simulink model "Cognata_Amp_Tobi_split1"  (R2020a)
settings: Solver=ode45  StartTime=0.0  StopTime=inf  RelTol=1e-3
model workspace (MAT data in the model file):
  cfg_native : object (value not decoded)
  en_add_channels = 1
  host_ip = 2130706433
  host_port = 50223
  local_ip = 2130706433
  local_port = 50224
  num_en_channels = 32
  num_samples = 1
  sample_rate = 250
  serial_number = 'NB-2015.10.93'
undefined symbols (not defined in the file or in its folder): A1, A104210, A138674, A141395, A30722, C1, C30722, currentCFG_Cognata_Amp_Tobi_split_UB, D1, D104210, I1, J138674, O141395, UB, W1, W104210
libraries: robotlib x18, gtecHighspeedLib x16, dspstat3 x2, simulink x2, TobiiEyeTrackerLib x1, gUSBamplib x1
settings Model: ModifiedByFormat=g.tec  Creator=g.tec medical engineering  LastModifiedBy=g.tec
settings DataIOCC: LimitDataPoints=on  SaveFormat=Array  ReturnWorkspaceOutputs=off
settings OptimizationCC: BlockReduction=off  BooleanDataType=off  LifeSpan=inf
settings DebuggingCC: SaveWithParameterizedLinksMsg=none  UnderspecifiedInitializationDetection=Classic  MergeDetectMultiDrivingBlocksExec=none  SignalResolutionControl=TryResolveAllWithWarning  FrameProcessingCompatibilityMsg=none  SFUnexpectedBacktrackingDiag=warning  SFNoUnconditionalDefaultTransitionDiag=warning  SFExecutionAtInitializationDiag=none  ArithmeticOperatorsInVariantConditions=warning
settings HardwareCC: ProdBitPerPointer=32  ProdBitPerSizeT=32  ProdBitPerPtrDiffT=32  ProdLargestAtomicFloat=None  ProdIntDivRoundTo=Undefined  ProdEndianess=Unspecified  ProdWordSize=32  ProdHWDeviceType=32-bit Generic  TargetUnknown=on
settings ModelReferenceCC: PropagateSignalLabelsOutOfModel=off
settings SFSimCC: SimUseLocalCustomCode=off  CustomCodeUndefinedFunction=UseInterfaceOnly
settings RTWCC: RTWUseLocalCustomCode=off
settings CodeAppCC: StateflowObjectComments=on
settings GRTTargetCC: TargetLangStandard=C89/C90 (ANSI)
settings ConfigComp: CovMetricSettings=dw  CovHtmlReporting=on  CovSaveCumulativeToWorkspaceVar=on  CovSaveSingleToWorkspaceVar=on  CovExternalEMLEnable=off

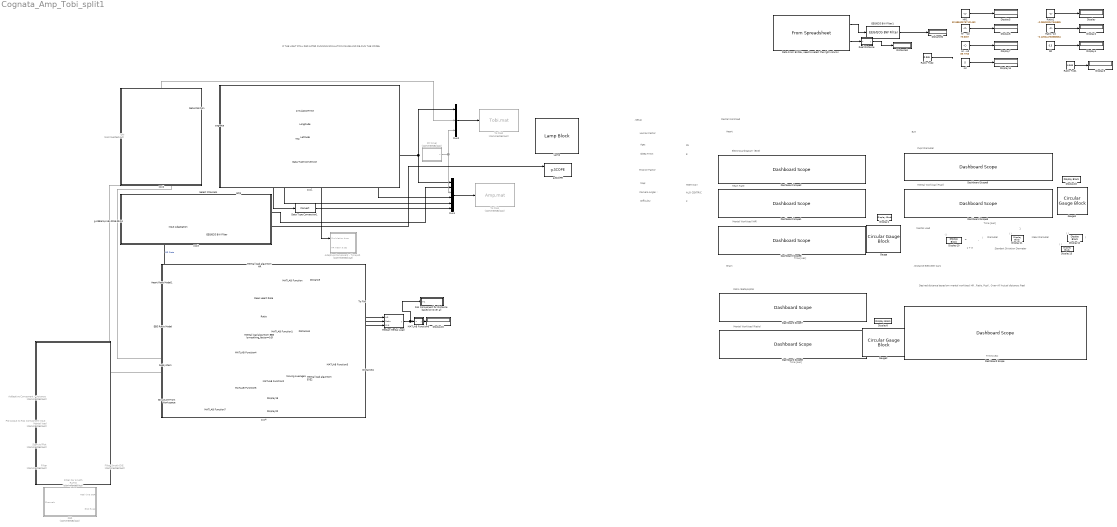
== system Cognata_Amp_Tobi_split1 ==
  note: Mental Load
  note: IF THE LIGHT STILL RED AFTER
      | RUNNING SIMULATION PAUSE AND RE-RUN THE MODEL
  note: Mission Factor
  note: Mental Workload
  note: Difficulty:
  note: Age:
  note: Brain
  note: ALO CENTRIC
  note: . Setup
  note: . Distance Between Cars
  note: Heart
  note: HIGH WAY
  note: Sleep Time:
  note: Camera Angle: :
  note: Human Factor
  note: Map:
  note: Electrocardiogram (ECG)
  note: Mental Workload (HR)
  note: Heart Rate
  note: Ratio (Beta/Alpha)
  note: Time [sec]
  note: Mental Workload (Ratio)
  note: Desired distance based om mental worklaod:
      | HR , Ratio, Pupil , Over-All
      |
      | Actual distance: Real
  note: Time [sec]
  note: 25
  note: 8
  note: 2
  note: Eye
  note: Pupil Diameter
  note: Mental Workload (Pupil)
  note: Time [sec]
  note: Time [sec]
  note: ( )
  note: 1
  note: Diameter
  note: ( )
  note: Mean Diameter
  note: ( )
  note: Standart Diviation Diameter
  note: ( )
  note: 1 + e
  note: (
  note: )
  note: -
  note: =
  "Adaptive Component - Time/HR " : Subsystem  Commented=on
  Addaptive Component - Distance : Subsystem  Commented=on
  Dashboard Scope : DashboardScope  ShowInitialText=off  TimeSpan=10  Ymin=-1  Ymax=20  LegendPosition=Hide  ScaleAtStop=off
  Dashboard Scope1 : DashboardScope  TimeSpan=10  Ymin=0  Ymax=100  LegendPosition=Hide  ScaleAtStop=off
  Dashboard Scope2 : DashboardScope  TimeSpan=10  Ymin=-3000  Ymax=1000  LegendPosition=Hide  ScaleAtStop=off
  Dashboard Scope3 : DashboardScope  TimeSpan=10  Ymin=0  Ymax=1  LegendPosition=Hide  ScaleAtStop=off
  Dashboard Scope6 : DashboardScope  TimeSpan=10  Ymin=0  Ymax=1  LegendPosition=Hide  ScaleAtStop=off
  Dashboard Scope7 : DashboardScope  TimeSpan=10  Ymin=0  Ymax=0.5  LegendPosition=Hide  ScaleAtStop=off
  Dashboard Scope8 : DashboardScope  TimeSpan=10  Ymin=0  Ymax=1  LegendPosition=Hide  ScaleAtStop=off
  Dashboard Scope9 : DashboardScope  TimeSpan=10  Ymin=0  Ymax=5  LegendPosition=Hide  ScaleAtStop=off
  "Data From EXCEL, need to select the right column " : FromSpreadsheet  FileName=C:\Users\LAB-OREN3\Desktop\CognataData\Participants_DATA\Test\4\g.techAmp Data of A1_546053_COMBINED_CUBE_DELAY_50_TTC_15 at (12;30;7).xlsx  SheetName=גיליון1  Range=A1:A104210,D1:D104210,W1:W104210  SampleTime=0.001953125
  Data Type Conversion : DataTypeConversion
  Data Type Conversion1 : DataTypeConversion
  Display{,2..7,14..15,19..20} (11 alike) : Display
  Display{1,8,10..11,13,16} (6 alike) : DisplayBlock  LabelPosition=Hide  Format=bank  Transparency=1
  Display12 : DisplayBlock  LabelPosition=Hide  Format=bank  Transparency=1  Layout=Fill available space
  Distance{,1..4} (5 alike) : Display
  ECG : MATLAB Function  TreatAsAtomicUnit=on
  EEG Ratio Model : Subsystem
  EEG/ECG BW Filter : gtecHighspeedLib/EEG//ECG BW Filter  Order=6  LowerFreq=0.1  UpperFreq=30  SampFreq=512
      settings: SourceProductName=g.HIsys Library
  EEG/ECG BW Filter1 : gtecHighspeedLib/EEG//ECG BW Filter  Order=6  LowerFreq=0.1  UpperFreq=30  SampFreq=512
      settings: SourceProductName=g.HIsys Library
  Filter : Subsystem  Commented=on
  Filter For smoth RATIO : Subsystem  Commented=on
  Filter Smoth EYE : Subsystem  Commented=on
  GSR : Subsystem  Commented=on
  Gauge : CircularGaugeBlock  LabelPosition=Hide  ScaleMax=1  TickInterval=0.2
  Gauge1 : CircularGaugeBlock  LabelPosition=Hide  ScaleMax=1  TickInterval=0.2
  Gauge2 : CircularGaugeBlock  LabelPosition=Hide  ScaleMax=1  TickInterval=0.2
  Gaze Position : Display
  HR1 : Constant  Value=82.688405797101450  VectorParams1D=off  SampleTime=0.5
  Heart Rate Model1 : ModelReference  ModelNameDialog=Heart_Rate_Model_Test  SimulationMode=Normal  ModelReferenceVersion=2.18.00
  Hr   -sd : Constant  Value=75.6007  SampleTime=0.5
  Hr - sd : Constant  Value=89.7753  SampleTime=0.5
  Input Adaptation : Subsystem
  Lamp : LampBlock
  Latitude : Display
  Longitude : Display
  MATLAB Function : MATLAB Function  TreatAsAtomicUnit=on
  MATLAB Function1 : MATLAB Function  TreatAsAtomicUnit=on
  MATLAB Function2 : MATLAB Function  TreatAsAtomicUnit=on
  MATLAB Function3 : MATLAB Function  TreatAsAtomicUnit=on
  MATLAB Function4 : MATLAB Function  TreatAsAtomicUnit=on
  MATLAB Function5 : MATLAB Function  TreatAsAtomicUnit=on
  MATLAB Function6 : MATLAB Function  TreatAsAtomicUnit=on
  MATLAB Function7 : MATLAB Function  TreatAsAtomicUnit=on
  "Mean Heart Rate " : Display
  Median Mental Load : MATLAB Function  TreatAsAtomicUnit=on
  "Mental load alguritom EEG (smoothing_factor=0.5) " : MATLAB Function  TreatAsAtomicUnit=on
  Mental load alguritom EYE2 : MATLAB Function  TreatAsAtomicUnit=on
  Mental load alguritom HR : MATLAB Function  TreatAsAtomicUnit=on
  Moving Average1 : dspstat3/Moving Average  Method=Sliding window  ForgettingFactorPort=off  SpecifyWindowLength=on  WindowLength=512  ForgettingFactor=0.9  SimulateUsing=Code generation
  Mux1 : Mux  Inputs=6
  Mux2 : Mux  Inputs=3
  PC timer : MATLAB Function  Commented=on  TreatAsAtomicUnit=on
  PID output to Ros Component input Mental load : Subsystem  Commented=on
  Ratio : Display
  Ratio +sd1 : Constant  Value=4.644  SampleTime=0.5
  Ratio +sd2 : Constant  Value=0.345  SampleTime=0.5
  Ratio -sd : Constant  Value=-0.125044783588084  SampleTime=0.5
  Ratio1 : Constant  Value=-0.086230047345885  VectorParams1D=off  SampleTime=0.5
  Real Distance : MATLAB Function  TreatAsAtomicUnit=on
  Ros Component for Distance based on Over all : Subsystem
  SD : Constant  Value=0.3  SampleTime=0.5
  Select Channels : gtecHighspeedLib/Select Channels  selectedchannels=[2]  totalchannels=14
      settings: SourceProductName=g.HIsys Library
  Sigmuid Plot : MATLAB Function  Commented=on  TreatAsAtomicUnit=on
  Structure From Workspace : FromWorkspace  VariableName=wave
  Subsystem : Subsystem
  TTC : Display
  To File : ToFile  Filename=Avrage.mat  MatrixName=Avrage
  To File1 : ToFile  Commented=on  Filename=Amp.mat  MatrixName=Ampdata
  To File2 : ToFile  Commented=on  Filename=Tobi.mat  MatrixName=Tobidata
  Tobi : Subsystem  Commented=on
  cognata : Subsystem
  g.SCOPE : gtecHighspeedLib/g.SCOPE
      settings: SourceProductName=g.HIsys Library
  g.USBamp UB-2015.09.13 : gUSBamplib/g.USBamp  cfg=currentCFG_Cognata_Amp_Tobi_split_UB-2015.09.13.cfg  snr=UB-2015.09.13
      settings: SourceProductName=g.USBamp
  sd : Constant  Value=5  SampleTime=0.5
  simulationTime : Display
  zzz1 : Subsystem  TreatAsAtomicUnit=on
      settings: OpenFcn=% no-op
      mask Display: disp('')
  zzz2 : Subsystem  TreatAsAtomicUnit=on
      settings: OpenFcn=% no-op
      mask Display: disp('')
  zzz3 : Subsystem  TreatAsAtomicUnit=on
      settings: OpenFcn=% no-op
      mask Display: disp('')
  zzz4 : Subsystem  TreatAsAtomicUnit=on
      settings: OpenFcn=% no-op
      mask Display: disp('')
  zzz5 : Subsystem  TreatAsAtomicUnit=on
      settings: OpenFcn=% no-op
      mask Display: disp('')
  wires:
  Tobi/2(Sum) -> Mux2/2
  Input Adaptation/1(Out) -> Mux1/2, EEG/ECG BW Filter/1
  Mux1/1 -> To File1/1
  Data Type Conversion/1 -> Mux2/1, Mux1/1, "Adaptive Component - Time/HR "/1(Simlulation time)
  g.USBamp UB-2015.09.13/1 -> Heart Rate Model1/1, EEG Ratio Model/1(Channels), Input Adaptation/1(In)  "EG Data"
  cognata/1(SimulationTime) -> Data Type Conversion/1, simulationTime/1
  Mux2/1 -> To File2/1
  Tobi/1(Gaze Pos) -> Gaze Position/1
  PC timer/1(z) -> Mux1/3, Mux2/3
  EEG/ECG BW Filter/1 -> Select Channels/1, g.SCOPE/1
  cognata/3(Latitude) -> Mux1/5, Latitude/1
  cognata/4(TTC) -> TTC/1, Data Type Conversion1/1
  cognata/2(Longitude) -> Mux1/4, Longitude/1
  Data Type Conversion1/1 -> Mux1/6
  MATLAB Function/1(y) -> Distance/1
  ECG/1(y) -> ?
  Select Channels/1 -> ECG/1(u)
  Mental load alguritom HR/1(y) -> Median Mental Load/1(HR), To File/1, MATLAB Function/1(u)
  "Mental load alguritom EEG (smoothing_factor=0.5) "/1(y) -> Median Mental Load/2(Ratio), MATLAB Function1/1(u)
  MATLAB Function1/1(y) -> Distance1/1
  "Data From EXCEL, need to select the right column "/1 -> EEG/ECG BW Filter1/1
  EEG/ECG BW Filter1/1 -> Distance2/1
  "Data From EXCEL, need to select the right column "/2 -> Real Distance/1(u)
  Ratio1/1 -> Display/1
  Ratio -sd/1 -> Display2/1
  SD/1 -> Display4/1
  Hr - sd/1 -> Display7/1
  Hr   -sd/1 -> Display6/1
  HR1/1 -> Display5/1
  Real Distance/1(y) -> Distance3/1
  sd/1 -> Display14/1
  Tobi/3(Pupil diameter Right Real-Time) -> Subsystem/1(Pupil diameter Right Real-Time)
  MATLAB Function2/1(y) -> Moving Average1/1
  Mental load alguritom EYE2/1(y) -> Median Mental Load/3(eye), MATLAB Function3/1(u)
  MATLAB Function3/1(y) -> Distance4/1
  Moving Average1/1 -> Mental load alguritom EYE2/1(u)
  MATLAB Function4/1(y) -> MATLAB Function2/1(u)
  MATLAB Function5/1(y) -> MATLAB Function2/2(Pupil_diameter_Left_Excel)
  Ratio +sd1/1 -> Display3/1
  Ratio +sd2/1 -> ?
  Tobi/4(Pupil diameter Left Real-Time1) -> Subsystem/2(Pupil diameter Left Real-Time1)
  Median Mental Load/1(y) -> Ros Component for Distance based on Over all/1(In1), MATLAB Function6/1(u)
  MATLAB Function6/1(y) -> Display15/1
  Structure From Workspace/1 -> MATLAB Function7/1(u)
  MATLAB Function7/2(z) -> MATLAB Function5/3(SD), MATLAB Function4/3(SD), Display20/1
  MATLAB Function7/1(y) -> MATLAB Function4/2(Mean), MATLAB Function5/2(Mean), Display19/1
  EEG Ratio Model/2(Real) -> Ratio/1, "Mental load alguritom EEG (smoothing_factor=0.5) "/1(u)
  Heart Rate Model1/1 -> "Mean Heart Rate "/1, Mental load alguritom HR/1(u)
  Subsystem/1(Real  time Right) -> MATLAB Function4/1(Pupil_diameter_Right)
  Subsystem/4(Real  time Left) -> MATLAB Function5/1(Pupil_diameter_Left)

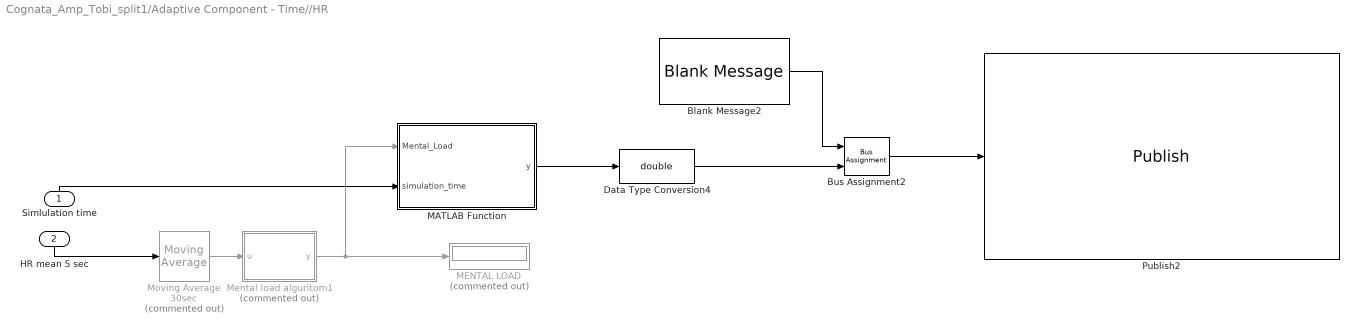
== system Cognata_Amp_Tobi_split1/Adaptive Component - Time//HR  ==
  Simlulation time : Inport
  HR mean 5 sec : Inport  Port=2
  Blank Message2 : robotlib/Blank Message  messageClass=Message  entityType=std_msgs/Float64  messageType=std_msgs/Float64  SampleTime=inf
  Bus Assignment2 : BusAssignment  AssignedSignals=Data
  Data Type Conversion4 : DataTypeConversion  OutDataTypeStr=double
  MATLAB Function : MATLAB Function  TreatAsAtomicUnit=on
  MENTAL LOAD : Display  Commented=on
  Mental load alguritom1 : MATLAB Function  Commented=on  TreatAsAtomicUnit=on
  Moving Average 30sec : dspstat3/Moving Average  Commented=on  Method=Sliding window  ForgettingFactorPort=off  SpecifyWindowLength=on  WindowLength=6000  ForgettingFactor=0.9  SimulateUsing=Code generation
  Publish2 : robotlib/Publish  topicSource=Specify your own  topic=/Test1  messageType=std_msgs/Float64  messageQueueLength=1
  wires:
  HR mean 5 sec/1 -> Moving Average 30sec/1
  MATLAB Function/1(y) -> Data Type Conversion4/1
  Moving Average 30sec/1 -> Mental load alguritom1/1(u)
  Simlulation time/1 -> MATLAB Function/2(simulation_time)
  Mental load alguritom1/1(y) -> MATLAB Function/1(Mental_Load), MENTAL LOAD/1
  Bus Assignment2/1 -> Publish2/1
  Blank Message2/1 -> Bus Assignment2/1
  Data Type Conversion4/1 -> Bus Assignment2/2

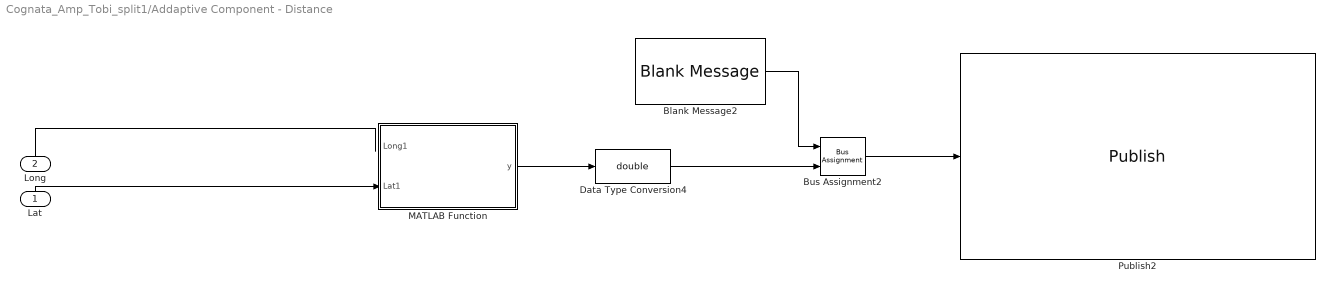
== system Cognata_Amp_Tobi_split1/Addaptive Component - Distance ==
  Lat : Inport
  Long : Inport  Port=2
  Blank Message2 : robotlib/Blank Message  SourceLibraryInfo=This block requires Robotics System Toolbox  messageType=std_msgs/Float64  SampleTime=inf
  Bus Assignment2 : BusAssignment  AssignedSignals=Data
  Data Type Conversion4 : DataTypeConversion  OutDataTypeStr=double
  MATLAB Function : MATLAB Function  TreatAsAtomicUnit=on
  Publish2 : robotlib/Publish  SourceLibraryInfo=This block requires Robotics System Toolbox  topicSource=Specify your own  topic=/Test1  messageType=std_msgs/Float64  messageQueueLength=1
  wires:
  MATLAB Function/1(y) -> Data Type Conversion4/1
  Lat/1 -> MATLAB Function/2(Lat1)
  Bus Assignment2/1 -> Publish2/1
  Blank Message2/1 -> Bus Assignment2/1
  Data Type Conversion4/1 -> Bus Assignment2/2
  Long/1 -> ?

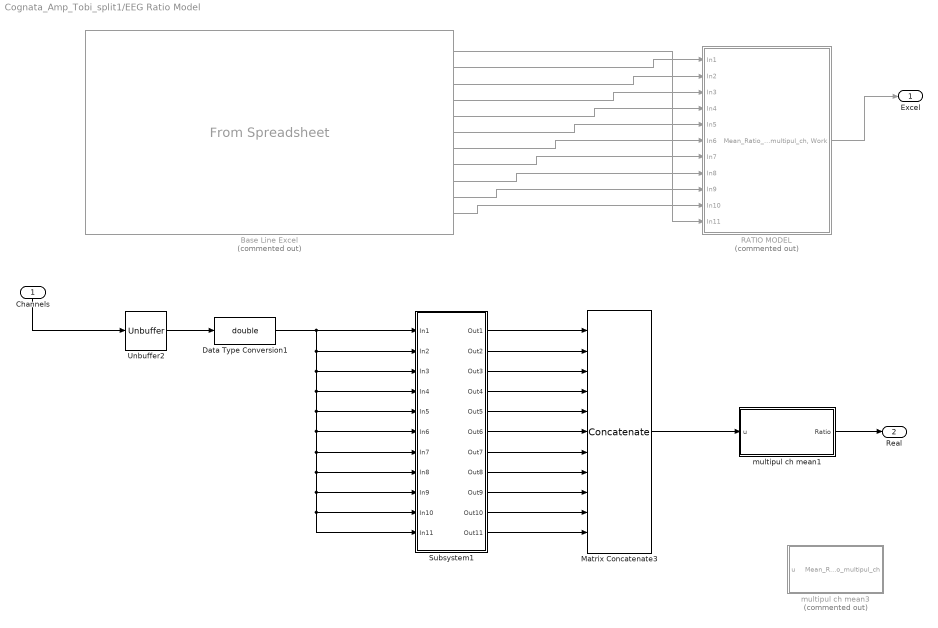
== system Cognata_Amp_Tobi_split1/EEG Ratio Model ==
  Channels : Inport
  Base Line Excel : FromSpreadsheet  Commented=on  FileName=C:\Users\LAB-OREN3\Downloads\1\g.techAmp Data of A2_535986_COMBINED_CUBE_DELAY_50_TTC_15 at (15;28;36).xlsx  SheetName=גיליון1  Range=A1:A141395,E1:O141395  SampleTime=0.001953125
  Data Type Conversion1 : DataTypeConversion  OutDataTypeStr=double
  Matrix Concatenate3 : Concatenate  NumInputs=11  Mode=Multidimensional array  ConcatenateDimension=2
  RATIO MODEL : Subsystem  Commented=on
  Subsystem1 : Subsystem
  Unbuffer2 : Unbuffer
  multipul ch mean1 : MATLAB Function  TreatAsAtomicUnit=on
  multipul ch mean3 : MATLAB Function  Commented=on  TreatAsAtomicUnit=on
  Excel : Outport
  Real : Outport  Port=2
  wires:
  Base Line Excel/1 -> RATIO MODEL/11(In11)
  Base Line Excel/6 -> RATIO MODEL/5(In5)
  Base Line Excel/7 -> RATIO MODEL/6(In6)
  Base Line Excel/2 -> RATIO MODEL/1(In1)
  Base Line Excel/11 -> RATIO MODEL/10(In10)
  Base Line Excel/3 -> RATIO MODEL/2(In2)
  Base Line Excel/5 -> RATIO MODEL/4(In4)
  Base Line Excel/4 -> RATIO MODEL/3(In3)
  Base Line Excel/8 -> RATIO MODEL/7(In7)
  Base Line Excel/10 -> RATIO MODEL/9(In9)
  Base Line Excel/9 -> RATIO MODEL/8(In8)
  Subsystem1/6(Out6) -> Matrix Concatenate3/6
  Subsystem1/2(Out2) -> Matrix Concatenate3/2
  Subsystem1/1(Out1) -> Matrix Concatenate3/1
  Subsystem1/8(Out8) -> Matrix Concatenate3/8
  Data Type Conversion1/1 -> Subsystem1/1(In1), Subsystem1/3(In3), Subsystem1/4(In4), Subsystem1/11(In11), Subsystem1/10(In10), Subsystem1/9(In9), Subsystem1/8(In8), Subsystem1/7(In7), Subsystem1/6(In6), Subsystem1/5(In5), Subsystem1/2(In2)
  Subsystem1/4(Out4) -> Matrix Concatenate3/4
  Subsystem1/5(Out5) -> Matrix Concatenate3/5
  Subsystem1/10(Out10) -> Matrix Concatenate3/10
  Subsystem1/9(Out9) -> Matrix Concatenate3/9
  Subsystem1/11(Out11) -> Matrix Concatenate3/11
  Matrix Concatenate3/1 -> multipul ch mean1/1(u)
  Unbuffer2/1 -> Data Type Conversion1/1
  Subsystem1/7(Out7) -> Matrix Concatenate3/7
  Subsystem1/3(Out3) -> Matrix Concatenate3/3
  Channels/1 -> Unbuffer2/1
  RATIO MODEL/1("Mean_Ratio_multipul_ch, Work") -> Excel/1
  multipul ch mean1/1(Ratio) -> Real/1

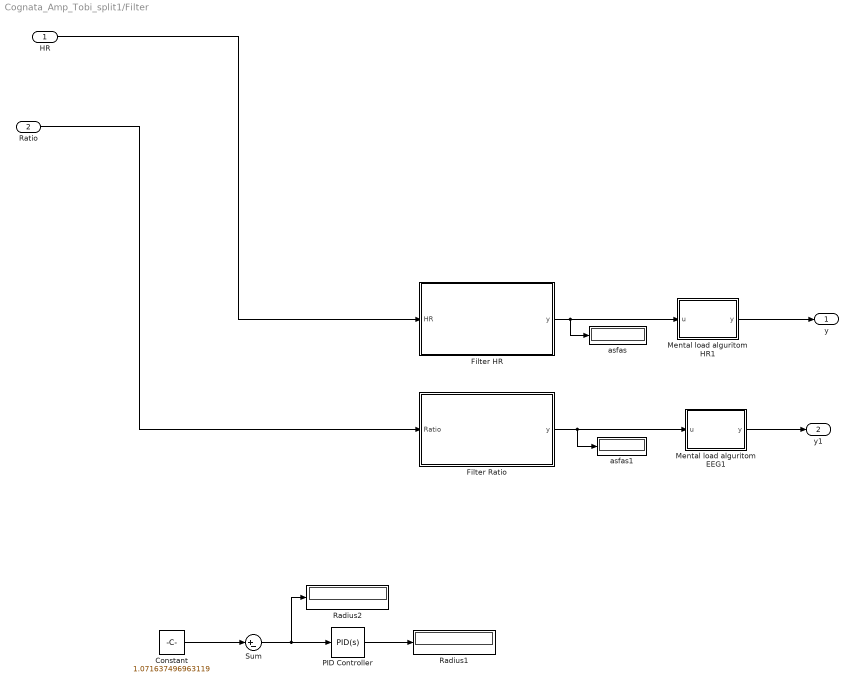
== system Cognata_Amp_Tobi_split1/Filter ==
  HR : Inport
  Ratio : Inport  Port=2
  Constant : Constant  Value=1.071637496963119
  Filter HR : MATLAB Function  TreatAsAtomicUnit=on
  Filter Ratio : MATLAB Function  TreatAsAtomicUnit=on
  Mental load alguritom EEG1 : MATLAB Function  TreatAsAtomicUnit=on
  Mental load alguritom HR1 : MATLAB Function  TreatAsAtomicUnit=on
  PID Controller : simulink/Continuous/PID Controller  Controller=PID  Form=Parallel  TimeDomain=Continuous-time  UseExternalTs=off  SampleTime=-1  IntegratorMethod=Forward Euler  FilterMethod=Forward Euler  ControllerParametersSource=internal  P=0  I=5  D=0  UseFilter=on  N=100  TunerSelectOption=Transfer Function Based (PID Tuner App)  InitialConditionSource=internal  InitialConditionForIntegrator=0  InitialConditionForFilter=0  DifferentiatorICPrevScaledInput=0  ExternalReset=none  TrackingMode=off  Kt=1  LimitOutput=off  UpperSaturationLimit=inf  LowerSaturationLimit=-inf  LinearizeAsGain=on  AntiWindupMode=none  Kb=1  POutMin=[]  POutMax=[]  IOutMin=[]  IOutMax=[]  DOutMin=[]  DOutMax=[]  NOutMin=[]  NOutMax=[]  SumOutMin=[]  SumOutMax=[]  SaturationOutMin=[]  SaturationOutMax=[]  PParamMin=[]  PParamMax=[]  IParamMin=[]  IParamMax=[]  DParamMin=[]  DParamMax=[]  NParamMin=[]  NParamMax=[]  KbParamMin=[]  KbParamMax=[]  KtParamMin=[]  KtParamMax=[]  KbOutMin=[]  KbOutMax=[]  KtOutMin=[]  KtOutMax=[]  IntegratorOutMin=[]  IntegratorOutMax=[]  FilterOutMin=[]  FilterOutMax=[]  SumI1OutMin=[]  SumI1OutMax=[]  SumI2OutMin=[]  SumI2OutMax=[]  SumI3OutMin=[]  SumI3OutMax=[]  SumI4OutMin=[]  SumI4OutMax=[]  SumDOutMin=[]  SumDOutMax=[]  DifferentiatorOutMin=[]  DifferentiatorOutMax=[]  FilterDiffOutCoefMin=[]  FilterDiffOutCoefMax=[]  ReciprocalOutMin=[]  ReciprocalOutMax=[]  SumDenOutMin=[]  SumDenOutMax=[]  SumNumOutMin=[]  SumNumOutMax=[]  DivideOutMin=[]  DivideOutMax=[]  UdiffTsProdOutMin=[]  UdiffTsProdOutMax=[]  NTsProdOutMin=[]  NTsProdOutMax=[]  UintegralTsProdOutMin=[]  UintegralTsProdOutMax=[]  UngainTsProdOutMin=[]  UngainTsProdOutMax=[]  IntegratorContinuousStateAttributes=''  IntegratorStateMustResolveToSignalObject=off  IntegratorRTWStateStorageClass=Auto  FilterContinuousStateAttributes=''  FilterStateMustResolveToSignalObject=off  FilterRTWStateStorageClass=Auto  ParallelPVariant=InternalParameters  IdealPVariant=Disabled  IVariant=InternalParameters  DVariant=InternalParameters  IntegratorVariant=Continuous  SatVariant=Disabled  AWVariant=Passthrough  PCopyVariant=Disabled  TRVariant=Disabled  FdbkBlocksVariant=Forward  IdealPFdbkVariant=Disabled  SatFdbkVariant=Disabled  DerivativeFilterVariant=ContFilter  NVariant=InternalParameters  NCopyVariant=Disabled  FilterICVariant=InternalICsFilter  IntegratorICVariant=InternalICs  ExternalResetVariant=Disabled  TRSumVariant=Passthrough  SumFdbkVariant=Disabled  SumVariant=Sum_PID  TsampFilterVariant=InternalTs  TsampNgainVariant=Passthrough  TsampIntegralVariant=Passthrough
  Radius1 : Display
  Radius2 : Display
  Sum : Sum  Inputs=|+-
  asfas : Display
  asfas1 : Display
  y : Outport
  y1 : Outport  Port=2
  wires:
  Filter Ratio/1(y) -> Mental load alguritom EEG1/1(u), asfas1/1
  Filter HR/1(y) -> Mental load alguritom HR1/1(u), asfas/1
  Mental load alguritom EEG1/1(y) -> y1/1
  HR/1 -> Filter HR/1(HR)
  Ratio/1 -> Filter Ratio/1(Ratio)
  Mental load alguritom HR1/1(y) -> y/1
  Constant/1 -> Sum/1
  Sum/1 -> Radius2/1, PID Controller/1
  PID Controller/1 -> Radius1/1
  ? -> Sum/2

== system Cognata_Amp_Tobi_split1/Filter For smoth RATIO ==
  u : Inport
  MATLAB Function2 : MATLAB Function  TreatAsAtomicUnit=on
  MATLAB Function4 : MATLAB Function  TreatAsAtomicUnit=on
  Mental load alguritom EEG1 : MATLAB Function  TreatAsAtomicUnit=on
  Radius3 : Display
  Transfer Fcn : TransferFcn  Numerator=1  Denominator=[1 1]
  y : Outport
  wires:
  Transfer Fcn/1 -> Mental load alguritom EEG1/1(u), Radius3/1
  MATLAB Function2/1(y) -> Transfer Fcn/1
  Mental load alguritom EEG1/1(y) -> MATLAB Function4/1(u)
  u/1 -> MATLAB Function2/1(u)
  MATLAB Function4/1(y) -> y/1

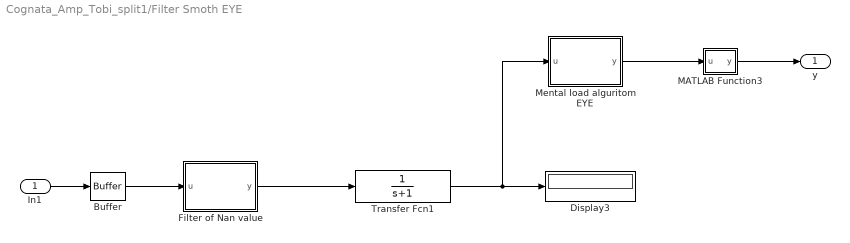
== system Cognata_Amp_Tobi_split1/Filter Smoth EYE ==
  In1 : Inport
  Buffer : Buffer  N=30  OutputFrames=off
  Display3 : Display
  Filter of Nan value : MATLAB Function  TreatAsAtomicUnit=on
  MATLAB Function3 : MATLAB Function  TreatAsAtomicUnit=on
  Mental load alguritom EYE : MATLAB Function  TreatAsAtomicUnit=on
  Transfer Fcn1 : TransferFcn  Numerator=1  Denominator=[1 1]
  y : Outport
  wires:
  Buffer/1 -> Filter of Nan value/1(u)
  Filter of Nan value/1(y) -> Transfer Fcn1/1
  Transfer Fcn1/1 -> Mental load alguritom EYE/1(u), Display3/1
  Mental load alguritom EYE/1(y) -> MATLAB Function3/1(u)
  MATLAB Function3/1(y) -> y/1
  In1/1 -> Buffer/1

== system Cognata_Amp_Tobi_split1/GSR ==
  Channels : Inport
  "Data From EXCEL, need to select the right column " : FromSpreadsheet  FileName=C:\Users\LAB-OREN3\Desktop\CognataData\Participants_DATA\Nadav_Test\Physiological\Stress\g.techAmp Data of Tese_GSR at (13;44;56).xlsx  SheetName=גיליון1  Range=A1:A30722,C1:C30722  SampleTime=0.001953125
  Data Type Conversion4 : DataTypeConversion  OutDataTypeStr=double
  Select Channels : gtecHighspeedLib/Select Channels  selectedchannels=[1]  totalchannels=14
      settings: SourceProductName=g.HIsys Library
  Unbuffer : Unbuffer
  Real time GSR : Outport
  GSR Excel : Outport  Port=2
  wires:
  Channels/1 -> Unbuffer/1
  Unbuffer/1 -> Data Type Conversion4/1
  Data Type Conversion4/1 -> Select Channels/1
  Select Channels/1 -> Real time GSR/1
  "Data From EXCEL, need to select the right column "/1 -> GSR Excel/1

== system Cognata_Amp_Tobi_split1/Input Adaptation ==
  In : Inport
  Data Type Conversion : DataTypeConversion  OutDataTypeStr=double
  Unbuffer : Unbuffer
  Out : Outport
  wires:
  In/1 -> Unbuffer/1
  Unbuffer/1 -> Data Type Conversion/1
  Data Type Conversion/1 -> Out/1

== system Cognata_Amp_Tobi_split1/PID output to Ros Component input Mental load ==
  In1 : Inport
  Constant : Constant
  PID Controller : simulink/Continuous/PID Controller  Controller=PID  Form=Parallel  TimeDomain=Continuous-time  UseExternalTs=off  SampleTime=-1  IntegratorMethod=Forward Euler  FilterMethod=Forward Euler  ControllerParametersSource=internal  P=1  I=1  D=0  UseFilter=on  N=100  TunerSelectOption=Transfer Function Based (PID Tuner App)  InitialConditionSource=internal  InitialConditionForIntegrator=0  InitialConditionForFilter=0  DifferentiatorICPrevScaledInput=0  ExternalReset=none  TrackingMode=off  Kt=1  LimitOutput=off  UpperSaturationLimit=inf  LowerSaturationLimit=-inf  LinearizeAsGain=on  AntiWindupMode=none  Kb=1  POutMin=[]  POutMax=[]  IOutMin=[]  IOutMax=[]  DOutMin=[]  DOutMax=[]  NOutMin=[]  NOutMax=[]  SumOutMin=[]  SumOutMax=[]  SaturationOutMin=[]  SaturationOutMax=[]  PParamMin=[]  PParamMax=[]  IParamMin=[]  IParamMax=[]  DParamMin=[]  DParamMax=[]  NParamMin=[]  NParamMax=[]  KbParamMin=[]  KbParamMax=[]  KtParamMin=[]  KtParamMax=[]  KbOutMin=[]  KbOutMax=[]  KtOutMin=[]  KtOutMax=[]  IntegratorOutMin=[]  IntegratorOutMax=[]  FilterOutMin=[]  FilterOutMax=[]  SumI1OutMin=[]  SumI1OutMax=[]  SumI2OutMin=[]  SumI2OutMax=[]  SumI3OutMin=[]  SumI3OutMax=[]  SumI4OutMin=[]  SumI4OutMax=[]  SumDOutMin=[]  SumDOutMax=[]  DifferentiatorOutMin=[]  DifferentiatorOutMax=[]  FilterDiffOutCoefMin=[]  FilterDiffOutCoefMax=[]  ReciprocalOutMin=[]  ReciprocalOutMax=[]  SumDenOutMin=[]  SumDenOutMax=[]  SumNumOutMin=[]  SumNumOutMax=[]  DivideOutMin=[]  DivideOutMax=[]  UdiffTsProdOutMin=[]  UdiffTsProdOutMax=[]  NTsProdOutMin=[]  NTsProdOutMax=[]  UintegralTsProdOutMin=[]  UintegralTsProdOutMax=[]  UngainTsProdOutMin=[]  UngainTsProdOutMax=[]  IntegratorContinuousStateAttributes=''  IntegratorStateMustResolveToSignalObject=off  IntegratorRTWStateStorageClass=Auto  FilterContinuousStateAttributes=''  FilterStateMustResolveToSignalObject=off  FilterRTWStateStorageClass=Auto  ParallelPVariant=InternalParameters  IdealPVariant=Disabled  IVariant=InternalParameters  DVariant=InternalParameters  IntegratorVariant=Continuous  SatVariant=Disabled  AWVariant=Passthrough  PCopyVariant=Disabled  TRVariant=Disabled  FdbkBlocksVariant=Forward  IdealPFdbkVariant=Disabled  SatFdbkVariant=Disabled  DerivativeFilterVariant=ContFilter  NVariant=InternalParameters  NCopyVariant=Disabled  FilterICVariant=InternalICsFilter  IntegratorICVariant=InternalICs  ExternalResetVariant=Disabled  TRSumVariant=Passthrough  SumFdbkVariant=Disabled  SumVariant=Sum_PID  TsampFilterVariant=InternalTs  TsampNgainVariant=Passthrough  TsampIntegralVariant=Passthrough
  Ros Component1 : Subsystem
  Sum : Sum  Inputs=+-
  wires:
  Sum/1 -> PID Controller/1
  Constant/1 -> Sum/1
  PID Controller/1 -> Ros Component1/1(In1)
  In1/1 -> Sum/2

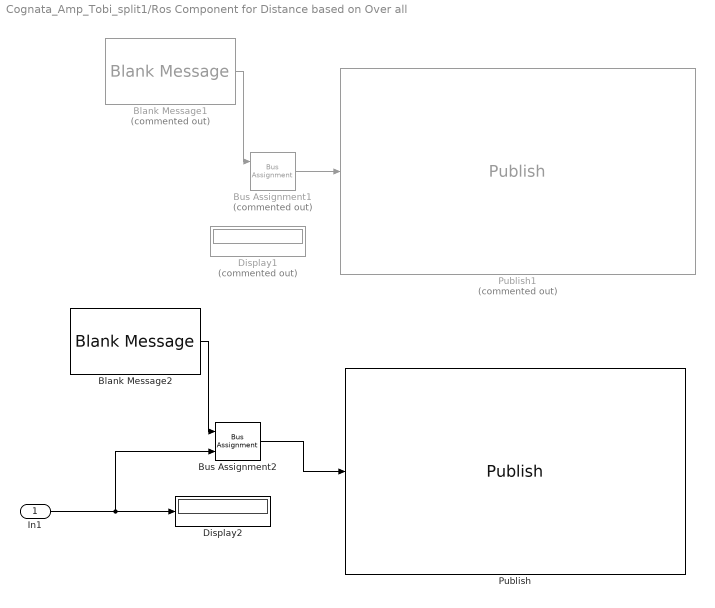
== system Cognata_Amp_Tobi_split1/Ros Component for Distance based on Over all ==
  In1 : Inport
  Blank Message1 : robotlib/Blank Message  Commented=on  messageClass=Message  entityType=std_msgs/Float64  messageType=std_msgs/Float64  SampleTime=inf
  Blank Message2 : robotlib/Blank Message  messageClass=Message  entityType=std_msgs/Float64  messageType=std_msgs/Float64  SampleTime=inf
  Bus Assignment1 : BusAssignment  Commented=on  AssignedSignals=Data
  Bus Assignment2 : BusAssignment  AssignedSignals=Data
  Display1 : Display  Commented=on
  Display2 : Display
  Publish : robotlib/Publish  topicSource=Specify your own  topic=/HR  messageType=std_msgs/Float64  messageQueueLength=1
  Publish1 : robotlib/Publish  Commented=on  topicSource=Specify your own  topic=/HR  messageType=std_msgs/Float64  messageQueueLength=1
  wires:
  Bus Assignment1/1 -> Publish1/1
  Blank Message1/1 -> Bus Assignment1/1
  In1/1 -> Bus Assignment2/2, Display2/1
  Blank Message2/1 -> Bus Assignment2/1
  Bus Assignment2/1 -> Publish/1

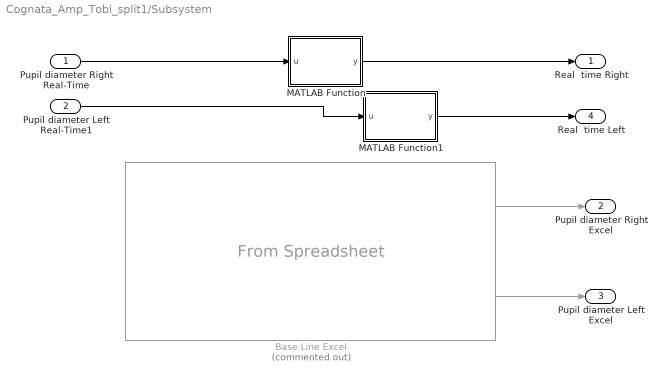
== system Cognata_Amp_Tobi_split1/Subsystem ==
  Pupil diameter Right Real-Time : Inport
  Pupil diameter Left Real-Time1 : Inport  Port=2
  Base Line Excel : FromSpreadsheet  Commented=on  FileName=C:\Users\LAB-OREN3\Downloads\1\Tobii Data of A2_535986_COMBINED_CUBE_DELAY_50_TTC_15 at (15;28;36).xlsx  SheetName=גיליון1  Range=A1:A138674,I1:J138674  SampleTime=0.001953125
  MATLAB Function : MATLAB Function  TreatAsAtomicUnit=on
  MATLAB Function1 : MATLAB Function  TreatAsAtomicUnit=on
  Real  time Right : Outport
  Pupil diameter Right Excel : Outport  Port=2
  Pupil diameter Left Excel : Outport  Port=3
  Real  time Left : Outport  Port=4
  wires:
  Base Line Excel/1 -> Pupil diameter Right Excel/1
  Base Line Excel/2 -> Pupil diameter Left Excel/1
  Pupil diameter Right Real-Time/1 -> MATLAB Function/1(u)
  Pupil diameter Left Real-Time1/1 -> MATLAB Function1/1(u)
  MATLAB Function/1(y) -> Real  time Right/1
  MATLAB Function1/1(y) -> Real  time Left/1

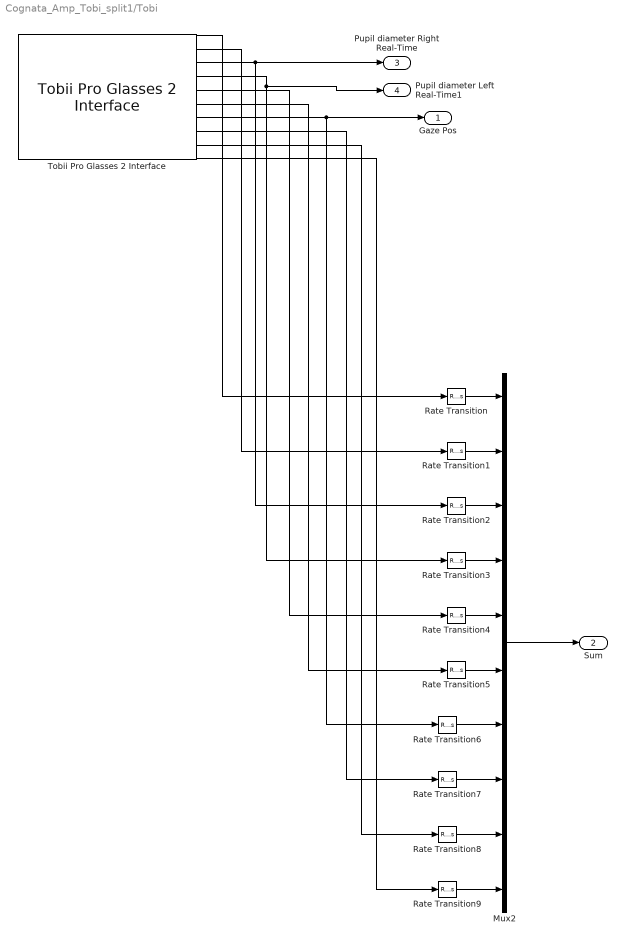
== system Cognata_Amp_Tobi_split1/Tobi ==
  Mux2 : Mux  Inputs=10
  Rate Transition{,1..9} (10 alike) : RateTransition  Deterministic=off  OutPortSampleTimeOpt=Inherit
  Tobii Pro Glasses 2 Interface : TobiiEyeTrackerLib/Tobii Pro Glasses 2 Interface  Key=0  pc_right=off  pc_left=off  pd_right=off  pd_left=off  gd_right=off  gd_left=off  gp=on  gp3=off  gy=off  ac=off
      settings: SourceProductName=g.EYEtracking Interface (Tobii Pro Glasses 2)
  Gaze Pos : Outport
  Sum : Outport  Port=2
  Pupil diameter Right Real-Time : Outport  Port=3
  Pupil diameter Left Real-Time1 : Outport  Port=4
  wires:
  Rate Transition1/1 -> Mux2/2
  Rate Transition9/1 -> Mux2/10
  Rate Transition6/1 -> Mux2/7
  Rate Transition7/1 -> Mux2/8
  Rate Transition8/1 -> Mux2/9
  Rate Transition/1 -> Mux2/1
  Rate Transition3/1 -> Mux2/4
  Rate Transition5/1 -> Mux2/6
  Rate Transition4/1 -> Mux2/5
  Mux2/1 -> Sum/1
  Rate Transition2/1 -> Mux2/3
  Tobii Pro Glasses 2 Interface/8 -> Rate Transition7/1
  Tobii Pro Glasses 2 Interface/2 -> Rate Transition1/1
  Tobii Pro Glasses 2 Interface/10 -> Rate Transition9/1
  Tobii Pro Glasses 2 Interface/9 -> Rate Transition8/1
  Tobii Pro Glasses 2 Interface/4 -> Rate Transition3/1, Pupil diameter Left Real-Time1/1
  Tobii Pro Glasses 2 Interface/7 -> Gaze Pos/1, Rate Transition6/1
  Tobii Pro Glasses 2 Interface/6 -> Rate Transition5/1
  Tobii Pro Glasses 2 Interface/1 -> Rate Transition/1
  Tobii Pro Glasses 2 Interface/5 -> Rate Transition4/1
  Tobii Pro Glasses 2 Interface/3 -> Rate Transition2/1, Pupil diameter Right Real-Time/1

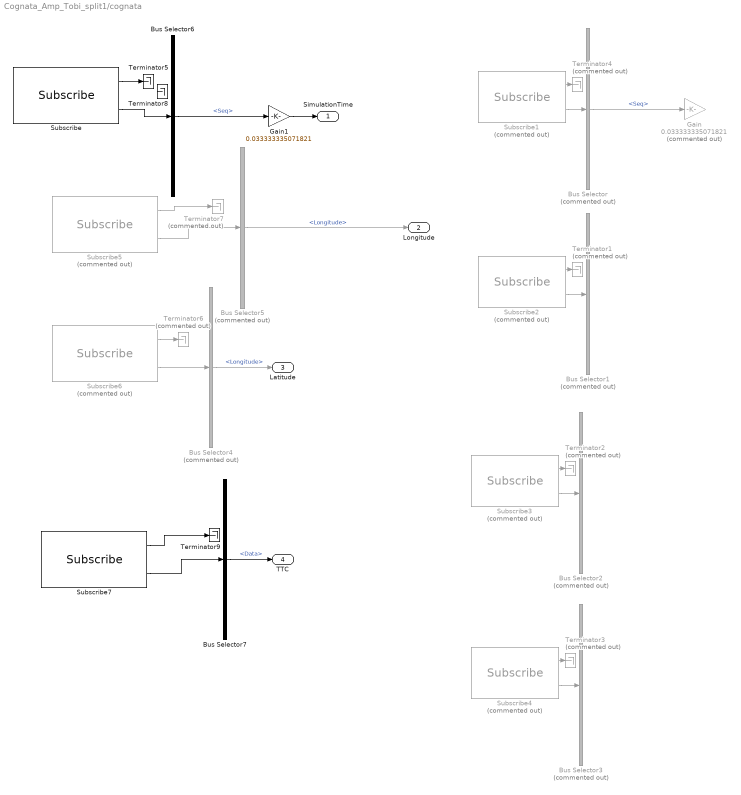
== system Cognata_Amp_Tobi_split1/cognata ==
  Bus Selector : BusSelector  Commented=on  OutputSignals=Header.Seq
  Bus Selector1 : BusSelector  Commented=on  OutputSignals=Longitude
  Bus Selector2 : BusSelector  Commented=on  OutputSignals=Latitude
  Bus Selector3 : BusSelector  Commented=on  OutputSignals=Data
  Bus Selector4 : BusSelector  Commented=on  OutputSignals=Longitude
  Bus Selector5 : BusSelector  Commented=on  OutputSignals=Longitude
  Bus Selector6 : BusSelector  OutputSignals=Header.Seq
  Bus Selector7 : BusSelector  OutputSignals=Data
  Gain : Gain  Commented=on  Gain=0.033333335071821
  Gain1 : Gain  Gain=0.033333335071821
  Subscribe : robotlib/Subscribe  topicSource=Specify your own  topic=/cognataSDK/GPS/info  messageType=sensor_msgs/NavSatFix  sampleTime=-1  messageQueueLength=1
  Subscribe1 : robotlib/Subscribe  Commented=on  topicSource=Specify your own  topic=/cognataSDK/GPS/info  messageType=sensor_msgs/NavSatFix  sampleTime=-1  messageQueueLength=10
  Subscribe2 : robotlib/Subscribe  Commented=on  topicSource=Specify your own  topic=/cognataSDK/GPS/info  messageType=sensor_msgs/NavSatFix  sampleTime=-1  messageQueueLength=10
  Subscribe3 : robotlib/Subscribe  Commented=on  topicSource=Specify your own  topic=/cognataSDK/GPS/info  messageType=sensor_msgs/NavSatFix  sampleTime=-1  messageQueueLength=10
  Subscribe4 : robotlib/Subscribe  Commented=on  topicSource=Specify your own  topic=/Distance_topic  messageType=std_msgs/Float32  sampleTime=-1  messageQueueLength=10
  Subscribe5 : robotlib/Subscribe  Commented=on  topicSource=Specify your own  topic=/cognataSDK/GPS/info  messageType=sensor_msgs/NavSatFix  sampleTime=-1  messageQueueLength=1
  Subscribe6 : robotlib/Subscribe  Commented=on  topicSource=Specify your own  topic=/cognataSDK/GPS/info  messageType=sensor_msgs/NavSatFix  sampleTime=-1  messageQueueLength=1
  Subscribe7 : robotlib/Subscribe  topicSource=Specify your own  topic=/Distance_topic  messageType=std_msgs/Float32  sampleTime=-1  messageQueueLength=1
  Terminator{1..4,6..7} (6 alike) : Terminator  Commented=on
  Terminator5 : Terminator
  Terminator8 : Terminator
  Terminator9 : Terminator
  SimulationTime : Outport
  Longitude : Outport  Port=2
  Latitude : Outport  Port=3
  TTC : Outport  Port=4
  wires:
  Bus Selector/1 -> Gain/1  "<Seq>"
  Subscribe1/2 -> Bus Selector/1
  Subscribe1/1 -> Terminator4/1
  Subscribe2/1 -> Terminator1/1
  Subscribe2/2 -> Bus Selector1/1
  Subscribe3/1 -> Terminator2/1
  Subscribe3/2 -> Bus Selector2/1
  Subscribe4/2 -> Bus Selector3/1
  Subscribe4/1 -> Terminator3/1
  Subscribe/1 -> Terminator5/1
  Bus Selector4/1 -> Latitude/1  "<Longitude>"
  Subscribe6/2 -> Bus Selector4/1
  Subscribe6/1 -> Terminator6/1
  Bus Selector5/1 -> Longitude/1  "<Longitude>"
  Subscribe5/2 -> Bus Selector5/1
  Subscribe5/1 -> Terminator7/1
  Subscribe/2 -> Bus Selector6/1
  Bus Selector6/1 -> Gain1/1  "<Seq>"
  Gain1/1 -> SimulationTime/1
  Subscribe7/2 -> Bus Selector7/1
  Subscribe7/1 -> Terminator9/1
  Bus Selector7/1 -> TTC/1  "<Data>"

== system Cognata_Amp_Tobi_split1/zzz1 ==

== system Cognata_Amp_Tobi_split1/zzz2 ==

== system Cognata_Amp_Tobi_split1/zzz3 ==

== system Cognata_Amp_Tobi_split1/zzz4 ==

== system Cognata_Amp_Tobi_split1/zzz5 ==

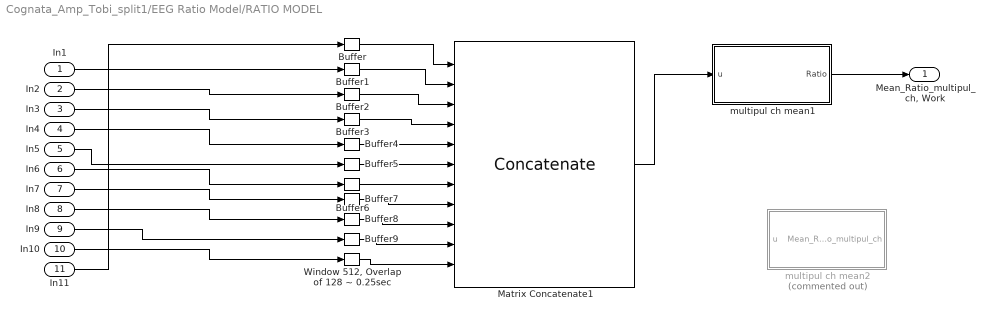
== system Cognata_Amp_Tobi_split1/EEG Ratio Model/RATIO MODEL ==
  In1 : Inport
  In2 : Inport  Port=2
  In3 : Inport  Port=3
  In4 : Inport  Port=4
  In5 : Inport  Port=5
  In6 : Inport  Port=6
  In7 : Inport  Port=7
  In8 : Inport  Port=8
  In9 : Inport  Port=9
  In10 : Inport  Port=10
  In11 : Inport  Port=11
  Buffer{,1..9} (10 alike) : Buffer  N=1536  V=1280  OutputFrames=off
  Matrix Concatenate1 : Concatenate  NumInputs=11  Mode=Multidimensional array  ConcatenateDimension=2
  "Window 512, Overlap of 128 ~ 0.25sec" : Buffer  N=1536  V=1280  OutputFrames=off
  multipul ch mean1 : MATLAB Function  TreatAsAtomicUnit=on
  multipul ch mean2 : MATLAB Function  Commented=on  TreatAsAtomicUnit=on
  "Mean_Ratio_multipul_ch, Work" : Outport
  wires:
  Buffer6/1 -> Matrix Concatenate1/7
  "Window 512, Overlap of 128 ~ 0.25sec"/1 -> Matrix Concatenate1/11
  Buffer3/1 -> Matrix Concatenate1/4
  Buffer2/1 -> Matrix Concatenate1/3
  Buffer4/1 -> Matrix Concatenate1/5
  Buffer5/1 -> Matrix Concatenate1/6
  Buffer/1 -> Matrix Concatenate1/1
  Buffer8/1 -> Matrix Concatenate1/9
  Buffer9/1 -> Matrix Concatenate1/10
  Buffer7/1 -> Matrix Concatenate1/8
  In7/1 -> Buffer7/1
  In10/1 -> "Window 512, Overlap of 128 ~ 0.25sec"/1
  Matrix Concatenate1/1 -> multipul ch mean1/1(u)
  Buffer1/1 -> Matrix Concatenate1/2
  In5/1 -> Buffer5/1
  In2/1 -> Buffer2/1
  In4/1 -> Buffer4/1
  In9/1 -> Buffer9/1
  In8/1 -> Buffer8/1
  In1/1 -> Buffer1/1
  In3/1 -> Buffer3/1
  In6/1 -> Buffer6/1
  In11/1 -> Buffer/1
  multipul ch mean1/1(Ratio) -> "Mean_Ratio_multipul_ch, Work"/1

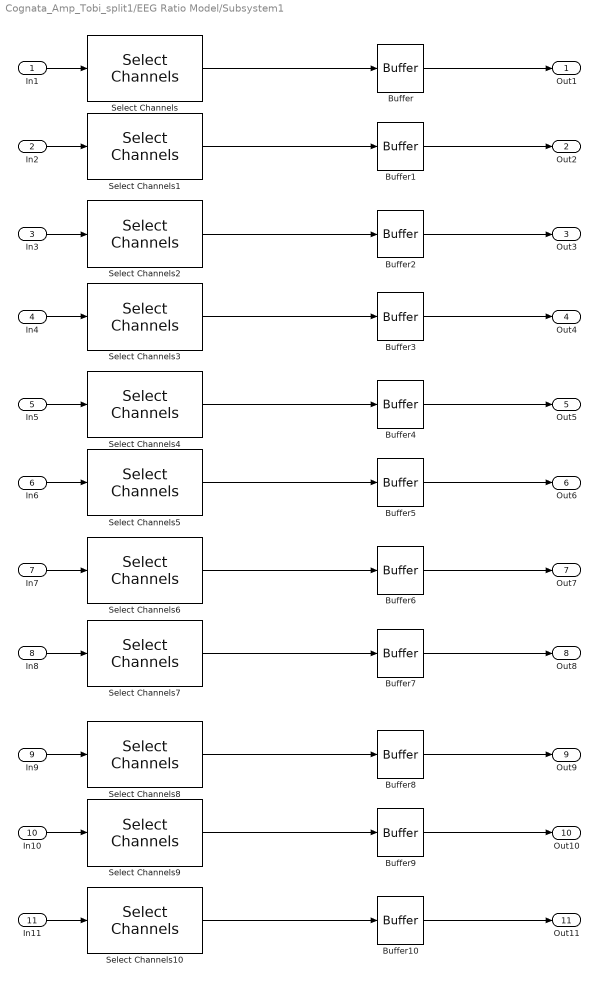
== system Cognata_Amp_Tobi_split1/EEG Ratio Model/Subsystem1 ==
  In1 : Inport
  In2 : Inport  Port=2
  In3 : Inport  Port=3
  In4 : Inport  Port=4
  In5 : Inport  Port=5
  In6 : Inport  Port=6
  In7 : Inport  Port=7
  In8 : Inport  Port=8
  In9 : Inport  Port=9
  In10 : Inport  Port=10
  In11 : Inport  Port=11
  Buffer{,1..10} (11 alike) : Buffer  N=1536  V=1280  OutputFrames=off
  Select Channels : gtecHighspeedLib/Select Channels  selectedchannels=[3]  totalchannels=14
      settings: SourceProductName=g.HIsys Library
  Select Channels1 : gtecHighspeedLib/Select Channels  selectedchannels=[4]  totalchannels=14
      settings: SourceProductName=g.HIsys Library
  Select Channels10 : gtecHighspeedLib/Select Channels  selectedchannels=[13]  totalchannels=14
      settings: SourceProductName=g.HIsys Library
  Select Channels2 : gtecHighspeedLib/Select Channels  selectedchannels=[5]  totalchannels=14
      settings: SourceProductName=g.HIsys Library
  Select Channels3 : gtecHighspeedLib/Select Channels  selectedchannels=[6]  totalchannels=14
      settings: SourceProductName=g.HIsys Library
  Select Channels4 : gtecHighspeedLib/Select Channels  selectedchannels=[7]  totalchannels=14
      settings: SourceProductName=g.HIsys Library
  Select Channels5 : gtecHighspeedLib/Select Channels  selectedchannels=[8]  totalchannels=14
      settings: SourceProductName=g.HIsys Library
  Select Channels6 : gtecHighspeedLib/Select Channels  selectedchannels=[9]  totalchannels=14
      settings: SourceProductName=g.HIsys Library
  Select Channels7 : gtecHighspeedLib/Select Channels  selectedchannels=[10]  totalchannels=14
      settings: SourceProductName=g.HIsys Library
  Select Channels8 : gtecHighspeedLib/Select Channels  selectedchannels=[11]  totalchannels=14
      settings: SourceProductName=g.HIsys Library
  Select Channels9 : gtecHighspeedLib/Select Channels  selectedchannels=[12]  totalchannels=14
      settings: SourceProductName=g.HIsys Library
  Out1 : Outport
  Out2 : Outport  Port=2
  Out3 : Outport  Port=3
  Out4 : Outport  Port=4
  Out5 : Outport  Port=5
  Out6 : Outport  Port=6
  Out7 : Outport  Port=7
  Out8 : Outport  Port=8
  Out9 : Outport  Port=9
  Out10 : Outport  Port=10
  Out11 : Outport  Port=11
  wires:
  In1/1 -> Select Channels/1
  Select Channels/1 -> Buffer/1
  In2/1 -> Select Channels1/1
  Select Channels1/1 -> Buffer1/1
  Buffer/1 -> Out1/1
  Buffer1/1 -> Out2/1
  Select Channels3/1 -> Buffer3/1
  Buffer3/1 -> Out4/1
  Select Channels2/1 -> Buffer2/1
  In4/1 -> Select Channels3/1
  In3/1 -> Select Channels2/1
  Buffer2/1 -> Out3/1
  Buffer6/1 -> Out7/1
  In8/1 -> Select Channels7/1
  In6/1 -> Select Channels5/1
  Select Channels7/1 -> Buffer7/1
  In5/1 -> Select Channels4/1
  Buffer4/1 -> Out5/1
  In7/1 -> Select Channels6/1
  Select Channels6/1 -> Buffer6/1
  Select Channels5/1 -> Buffer5/1
  Select Channels4/1 -> Buffer4/1
  Buffer7/1 -> Out8/1
  Buffer5/1 -> Out6/1
  In10/1 -> Select Channels9/1
  In9/1 -> Select Channels8/1
  Buffer10/1 -> Out11/1
  Buffer8/1 -> Out9/1
  Buffer9/1 -> Out10/1
  Select Channels9/1 -> Buffer9/1
  Select Channels10/1 -> Buffer10/1
  In11/1 -> Select Channels10/1
  Select Channels8/1 -> Buffer8/1

== system Cognata_Amp_Tobi_split1/PID output to Ros Component input Mental load/Ros Component1 ==
  In1 : Inport
  Blank Message1 : robotlib/Blank Message  SourceLibraryInfo=This block requires Robotics System Toolbox  messageType=std_msgs/Float64  SampleTime=inf
  Bus Assignment1 : BusAssignment  AssignedSignals=Data
  Display1 : Display
  Publish1 : robotlib/Publish  SourceLibraryInfo=This block requires Robotics System Toolbox  topicSource=Specify your own  topic=/HR  messageType=std_msgs/Float64  messageQueueLength=1
  wires:
  Blank Message1/1 -> Bus Assignment1/1
  Bus Assignment1/1 -> Publish1/1
  In1/1 -> Display1/1, Bus Assignment1/2

== matlab function Cognata_Amp_Tobi_split1/MATLAB Function1 ==
  data: u input; y output
function y = fcn(u)
%#codegen

y = (u*10)+10;

== matlab function Cognata_Amp_Tobi_split1/EEG Ratio Model/multipul ch mean3 ==
  data: u input; Mean_Ratio_multipul_ch output
function Mean_Ratio_multipul_ch = EEG_Stress_Ratio(u)

   coder.extrinsic('pwelch');
   coder.extrinsic('table2array');
   sampling_rate = 512;
   % On a 512 sampling rate we should have 129 freqwencies: to Obtain the Welch PSD estimate dividing the signal into segments 132 samples in length. The signal segments are multiplied by a Hamming window 132 samples in length. The number of overlapped samples is not specified, so it is set to 132/2 = 66. The DFT length is 256 points, yielding a frequency resolution of  rad/sample. Because the signal is real-valued, the PSD estimate is one-sided and there are 256/2+1 = 129 points. Plot the PSD as a function of normalized frequency.
   % 
   number_of_frquencies = (size(u, 1)/4)+1;
   psd = zeros(number_of_frquencies,1);
   frequencies = zeros(number_of_frquencies,1);
  
   %initialize an array to store the stress scores for each channel
   stress_scores = zeros(size(u, 2), 1);
   
   
       for i = 1:size(u, 2)
            
           %extract for current channel
           channel_data = u(:, i);
            
           % Calculate the power spectral density (PSD) of the EEG data
           [psd, frequencies] = pwelch(channel_data, [], [], [], sampling_rate);


           % Calculate the relative power in the alpha frequency band (8-12 Hz)
           alpha_power = sum(psd(frequencies >= 8 & frequencies <= 12)) / sum(psd);

           % Calculate the relative power in the beta frequency band (12-30 Hz)
           beta_power = sum(psd(frequencies >= 12 & frequencies <= 30)) / sum(psd);

           % Calculate the alpha/beta ratio for the current channel
%            alpha_beta_ratio = beta_power / alpha_power ;
             alpha_beta_ratio = log(beta_power) - log(alpha_power) ;


            stress_scores(i) = alpha_beta_ratio;
            
       end
  
 
    Mean_Ratio_multipul_ch = mean(stress_scores);
end

== matlab function Cognata_Amp_Tobi_split1/Filter/Filter Ratio ==
  data: Ratio input; y output
function y = fcn(Ratio)

    
    if Ratio >= -0.125
     y = -0.125;
    elseif Ratio <= -0.0474 
     y = -0.0474;
    else
    y =Ratio;
    end

   
end

== matlab function Cognata_Amp_Tobi_split1/MATLAB Function ==
  data: u input; y output
function y = fcn(u)
%#codegen

y = (u*10)+10;

== matlab function Cognata_Amp_Tobi_split1/Filter/Mental load alguritom EEG1 ==
  data: u input; y output
function y = fcn(u)

y= probability_of_metal_load_EEG(u);

end

== matlab function Cognata_Amp_Tobi_split1/Median Mental Load ==
  data: HR input; y output; Ratio input; eye input
function y = fcn(HR, Ratio, eye)

vac = [HR Ratio eye];
y = median(vac);

end

== matlab function Cognata_Amp_Tobi_split1/Subsystem/MATLAB Function ==
  data: u input; y output
function y = fcn(u)

y = u;

== matlab function Cognata_Amp_Tobi_split1/Filter For smoth RATIO/MATLAB Function2 ==
  data: u input; y output
function y = fcn(u)
    if isnan(u)
        y = 1.0;
    else 
        y=u;
    end
end

== matlab function Cognata_Amp_Tobi_split1/Filter Smoth EYE/Mental load alguritom EYE ==
  data: u input; y output
function y = fcn(u)

y= probability_of_metal_load_EYE(u);

end

== matlab function Cognata_Amp_Tobi_split1/Filter For smoth RATIO/Mental load alguritom EEG1 ==
  data: u input; y output
function y = fcn(u)

y= probability_of_metal_load_EEG(u);

end

== matlab function Cognata_Amp_Tobi_split1/Filter For smoth RATIO/MATLAB Function4 ==
  data: u input; y output
function y = fcn(u)
%#codegen

y = (u*10)+10;

== matlab function Cognata_Amp_Tobi_split1/Filter Smoth EYE/Filter of Nan value ==
  data: u input; y output
function y = fcn(u)

avg = mean(u);

y = avg;

== matlab function Cognata_Amp_Tobi_split1/Subsystem/MATLAB Function1 ==
  data: u input; y output
function y = fcn(u)

y = u;

== matlab function Cognata_Amp_Tobi_split1/PC timer ==
  data: z output
function z = fcn()
eml.extrinsic('clock'); 
t = [0,0,0,0,0,0];
t = clock;
k = t(1,4:6);
z = k';
end

== matlab function Cognata_Amp_Tobi_split1/Filter Smoth EYE/MATLAB Function3 ==
  data: u input; y output
function y = fcn(u)
%#codegen

y = (u*10)+10;

== matlab function Cognata_Amp_Tobi_split1/MATLAB Function6 ==
  data: u input; y output
function y = fcn(u)
%#codegen

y = (u*10)+10;

== matlab function Cognata_Amp_Tobi_split1/MATLAB Function7 ==
  data: u input; y output; z output
function [y,z]  = func(u)



y = u(1,1);
z = u(2,1);

== matlab function Cognata_Amp_Tobi_split1/MATLAB Function2 ==
  data: u input; y output; Pupil_diameter_Left_Excel input
function y = fcn(u, Pupil_diameter_Left_Excel)
 
    
y = (u+Pupil_diameter_Left_Excel)/2;

== matlab function Cognata_Amp_Tobi_split1/Mental load alguritom EYE2 ==
  data: u input; y output
function y = fcn(u)

y= probability_of_metal_load_EYE(u);

end

== matlab function Cognata_Amp_Tobi_split1/MATLAB Function3 ==
  data: u input; y output
function y = fcn(u)
%#codegen

y = (u*10)+10;

== matlab function Cognata_Amp_Tobi_split1/MATLAB Function4 ==
  data: Pupil_diameter_Right input; y output; Mean input; SD input
function y = fcn(Pupil_diameter_Right, Mean, SD)
    
  if Pupil_diameter_Right < 2.0 
      y = Mean-(2*SD);
  elseif Pupil_diameter_Right > 8.0
      y = Mean+(2*SD);
  else
      y = Pupil_diameter_Right;
  end
end

== matlab function Cognata_Amp_Tobi_split1/MATLAB Function5 ==
  data: Pupil_diameter_Left input; y output; Mean input; SD input
function y = fcn(Pupil_diameter_Left, Mean, SD)
    
  if Pupil_diameter_Left < 2.0 
      y = Mean-(2*SD);
  elseif Pupil_diameter_Left > 8.0
      y = Mean+(2*SD);
  else
      y = Pupil_diameter_Left;
  end
end

== matlab function Cognata_Amp_Tobi_split1/Adaptive Component - Time//HR /Mental load alguritom1 ==
  data: u input; y output
function y = fcn(u)

y= probability_of_mental_workload_30sec(u);

end

== matlab function Cognata_Amp_Tobi_split1/EEG Ratio Model/RATIO MODEL/multipul ch mean1 ==
  data: u input; Ratio output
function Ratio = EEG_Stress_Ratio(u)

Ratio= eeg_stress_ratio(u);


end

== matlab function Cognata_Amp_Tobi_split1/EEG Ratio Model/multipul ch mean1 ==
  data: u input; Ratio output
function Ratio = EEG_Stress_Ratio(u)

Ratio= eeg_stress_ratio(u);


end

== matlab function Cognata_Amp_Tobi_split1/Adaptive Component - Time//HR /MATLAB Function ==
  data: Mental_Load input; simulation_time input; y output
function y = fcn(Mental_Load, simulation_time)
%#codegen

%y = 0;% function output

%if  (30.0 < data )&&(data < 30.1)

decision_time=60.0;
if (decision_time < simulation_time )&&(decision_time+0.1 > simulation_time)% && (Mental_Load < 0.5)    
    
y = 1.0; % SEND MESSAGE

else
    
y = 0.0; % DONT SEND MESSAGE   

end

== matlab function Cognata_Amp_Tobi_split1/Mental load alguritom HR ==
  data: u input; y output
function y = fcn(u)

y= probability_of_mental_load_HR(u);

end

== matlab function Cognata_Amp_Tobi_split1/Addaptive Component - Distance/MATLAB Function ==
  data: Long1 input; Lat1 input; y output
function y = fcn(Long1, Lat1)
%#codegen

Stop_latitude_Point = 0.0;
Stop_longitude_Point = 0.0;

%y = 0;% function output
Distance_Between_Two_Cordinants_km = deg2km(distance(Long1,Lat1,48.17946869101,11.5851688385))
%if  (30.0 < data )&&(data < 30.1)


if (Distance_Between_Two_Cordinants_km < 0.050)% && (Mental_Load < 0.5)    
    
y = 1.0; % SEND MESSAGE

else
    
y = 0.0; % DONT SEND MESSAGE   

end

== matlab function Cognata_Amp_Tobi_split1/ECG ==
  data: u input; y output
function y = fcn(u)

y = u;

== matlab function Cognata_Amp_Tobi_split1/Mental load alguritom EEG (smoothing_factor=0.5)  ==
  data: u input; y output
function y = fcn(u)

y= probability_of_metal_load_EEG(u);

end

== matlab function Cognata_Amp_Tobi_split1/Filter/Filter HR ==
  data: HR input; y output
function y = fcn(HR)

    
    if HR >= 105.0
     y = 105.0;
    elseif HR <= 94.0 
     y = 94.0;
    else
    y =HR;
    end

   
end

== matlab function Cognata_Amp_Tobi_split1/Sigmuid Plot ==
  data: u input; g output
function g = fcn(u)

u = int16(u);

u = (u * 997) + 1.0;

u = int16(u);

x = linspace(-10, 10 ,1000); % vector of x

y = 1 ./ (1 + exp(-x));

% Set the range of x-values
% xlim([-10, 10]);  % range of ציר X


% Plot the function
% figure('MenuBar', 'none', 'ToolBar', 'none');
% fig = figure('Position', [50, 50, 100, 100]);
plot(x, y, 'color', 'red');
hold on


h = plot(x, y, 'o', 'MarkerIndices', u); 
% pause(0.44);
set(h, 'MarkerIndices', []);


g = u;

== matlab function Cognata_Amp_Tobi_split1/EEG Ratio Model/RATIO MODEL/multipul ch mean2 ==
  data: u input; Mean_Ratio_multipul_ch output
function Mean_Ratio_multipul_ch = EEG_Stress_Ratio(u)



    
   coder.extrinsic('pwelch');
   coder.extrinsic('table2array');
   sampling_rate = 512;
   psd = zeros(513,1);
   frequencies = zeros(513,1);
   
   
   % On a 512 sampling rate we should have 129 freqwencies: to Obtain the Welch PSD estimate dividing the signal into segments 132 samples in length. The signal segments are multiplied by a Hamming window 132 samples in length. The number of overlapped samples is not specified, so it is set to 132/2 = 66. The DFT length is 256 points, yielding a frequency resolution of  rad/sample. Because the signal is real-valued, the PSD estimate is one-sided and there are 256/2+1 = 129 points. Plot the PSD as a function of normalized frequency.
   % 
%    number_of_frquencies = (size(u, 1)/4)+1;
%    disp(number_of_frquencies);
%    psd = zeros(number_of_frquencies,1);
%    frequencies = zeros(number_of_frquencies,1);
  
   %initialize an array to store the stress scores for each channel
   stress_scores = zeros(size(u, 2), 1);
   
   
       for i = 1:size(u, 2)
           
%           u=table2array(u);
           %extract for current channel
           channel_data = u(:, i);
%            disp("Alex");
%            disp(class(channel_data));
%            disp(channel_data);
%            disp("Alex");
%            disp(size(channel_data));

            
           % Calculate the power spectral density (PSD) of the EEG data
           [psd, frequencies] = pwelch(channel_data, [], [], [], sampling_rate);
%             disp("psd test");
%             disp(psd);


           % Calculate the relative power in the alpha frequency band (8-12 Hz)
           alpha_power = sum(psd(frequencies >= 8 & frequencies <= 12));
%            disp("alpha_power");
%            disp(alpha_power);  
           
           % Calculate the relative power in the beta frequency band (12-30 Hz)
           beta_power = sum(psd(frequencies >= 12 & frequencies <= 30));
%            disp("beta_power");
%            disp(beta_power);  
           % Calculate the alpha/beta ratio for the current channel
%            alpha_beta_ratio = beta_power / alpha_power ;
             alpha_beta_ratio = log(beta_power/alpha_power) ;


            stress_scores(i) = alpha_beta_ratio;
            
            
       end
  
 
    Mean_Ratio_multipul_ch = mean(stress_scores);
end

== matlab function Cognata_Amp_Tobi_split1/Filter/Mental load alguritom HR1 ==
  data: u input; y output
function y = fcn(u)

y= probability_of_mental_howrkload(u);

end

== matlab function Cognata_Amp_Tobi_split1/Real Distance ==
  data: u input; y output
function y = fcn(u)

y = u;
